simulink model "spc_nonlinear_observer_extended"  (R2022b)
settings: Solver=VariableStepAuto  StartTime=0.0  StopTime=30  RelTol=1e-3
undefined symbols (not defined in the file): A, B, C, D, g, Ki, Kp, L, l, M, m
settings Model: Creator=CANER  LastModifiedBy=CANER

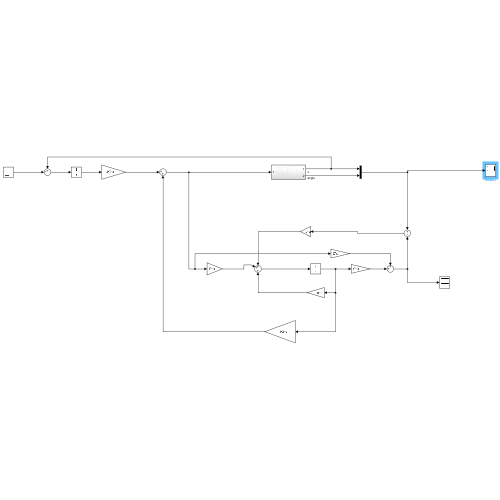
[thumbnail: Simulink's stored preview of the top-level diagram]
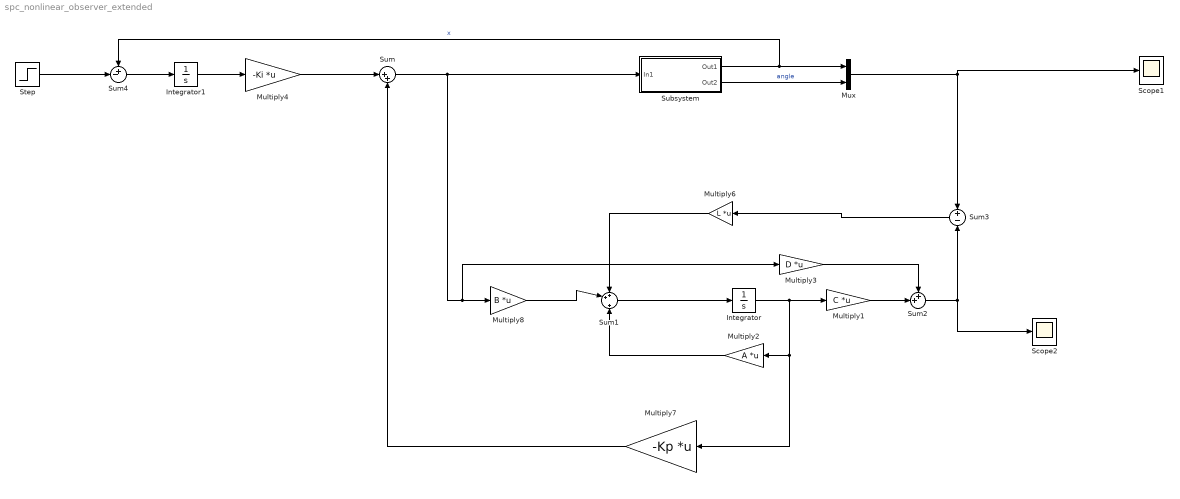
== system spc_nonlinear_observer_extended ==
  Integrator : Integrator
  Integrator1 : Integrator
  Multiply1 : Gain  Gain=C  Multiplication=Matrix(K*u)
  Multiply2 : Gain  Gain=A  Multiplication=Matrix(K*u)
  Multiply3 : Gain  Gain=D  Multiplication=Matrix(K*u)
  Multiply4 : Gain  Gain=-Ki  Multiplication=Matrix(K*u)
  Multiply6 : Gain  Gain=L  Multiplication=Matrix(K*u)
  Multiply7 : Gain  Gain=-Kp  Multiplication=Matrix(K*u)
  Multiply8 : Gain  Gain=B  Multiplication=Matrix(K*u)
  Mux : Mux  Inputs=2
  Scope1 : Scope
  Scope2 : Scope
  Step : Step  Time=0  SampleTime=0
  Subsystem : Subsystem
  Sum : Sum  Inputs=|++
  Sum1 : Sum  Inputs=++|+
  Sum2 : Sum  Inputs=++|
  Sum3 : Sum  Inputs=+|-
  Sum4 : Sum  Inputs=+-|
  wires:
  Multiply7/1 -> Sum/2
  Multiply6/1 -> Sum1/1
  Sum3/1 -> Multiply6/1
  Multiply8/1 -> Sum1/2
  Multiply2/1 -> Sum1/3
  Sum1/1 -> Integrator/1
  Integrator/1 -> Multiply7/1, Multiply2/1, Multiply1/1
  Sum2/1 -> Sum3/2, Scope2/1
  Sum/1 -> Subsystem/1(In1), Multiply3/1, Multiply8/1
  Subsystem/1(Out1) -> Sum4/1, Mux/1  "x"
  Multiply1/1 -> Sum2/2
  Multiply3/1 -> Sum2/1
  Mux/1 -> Sum3/1, Scope1/1
  Subsystem/2(Out2) -> Mux/2  "angle"
  Step/1 -> Sum4/2
  Multiply4/1 -> Sum/1
  Integrator1/1 -> Multiply4/1
  Sum4/1 -> Integrator1/1

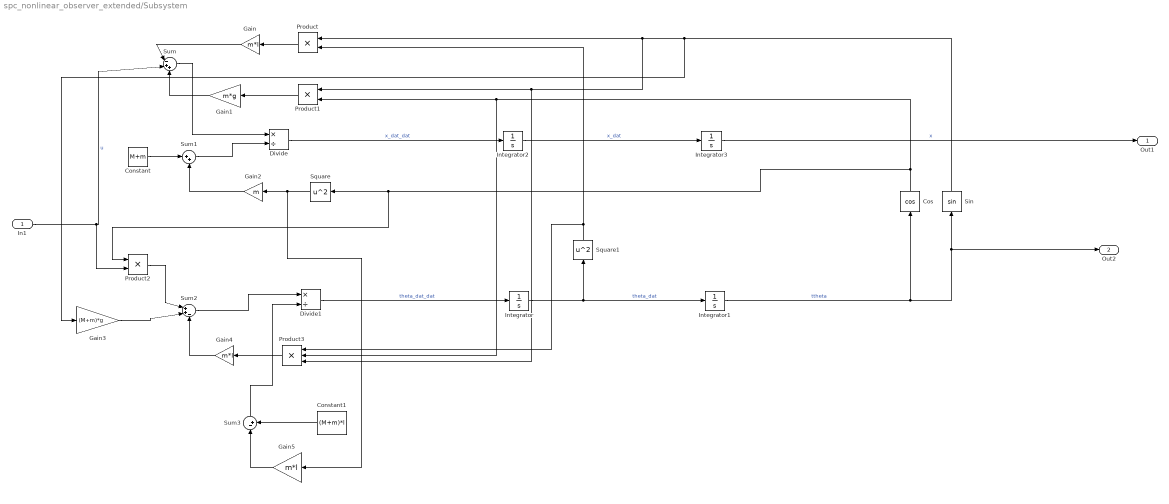
== system spc_nonlinear_observer_extended/Subsystem ==
  In1 : Inport
  Constant : Constant  Value=M+m
  Constant1 : Constant  Value=(M+m)*l
  Cos : Trigonometry  Operator=cos
  Divide : Product  Inputs=*/
  Divide1 : Product  Inputs=*/
  Gain : Gain  Gain=m*l
  Gain1 : Gain  Gain=m*g
  Gain2 : Gain  Gain=m
  Gain3 : Gain  Gain=(M+m)*g
  Gain4 : Gain  Gain=m*l
  Gain5 : Gain  Gain=m*l
  Integrator{,1..3} (4 alike) : Integrator
  Product : Product
  Product1 : Product
  Product2 : Product
  Product3 : Product  Inputs=3
  Sin : Trigonometry
  Square : Math  Operator=square
  Square1 : Math  Operator=square
  Sum : Sum  Inputs=|-++
  Sum1 : Sum  Inputs=|++
  Sum2 : Sum  Inputs=|++-
  Sum3 : Sum  Inputs=|-+
  Out1 : Outport
  Out2 : Outport  Port=2
  wires:
  Integrator/1 -> Integrator1/1, Square1/1  "theta_dat"
  Integrator2/1 -> Integrator3/1  "x_dat"
  Integrator3/1 -> Out1/1  "x"
  Divide/1 -> Integrator2/1  "x_dat_dat"
  Divide1/1 -> Integrator/1  "theta_dat_dat"
  Integrator1/1 -> Out2/1, Sin/1, Cos/1  "ttheta"
  In1/1 -> Product2/2, Sum/2  "u"
  Product/1 -> Gain/1
  Gain/1 -> Sum/1
  Gain1/1 -> Sum/3
  Cos/1 -> Product2/1, Square/1, Product3/2, Product1/2
  Product1/1 -> Gain1/1
  Sum/1 -> Divide/1
  Constant/1 -> Sum1/1
  Gain2/1 -> Sum1/2
  Square/1 -> Gain5/1, Gain2/1
  Sum1/1 -> Divide/2
  Product2/1 -> Sum2/1
  Sin/1 -> Gain3/1, Product3/3, Product1/1, Product/1
  Gain3/1 -> Sum2/2
  Gain4/1 -> Sum2/3
  Product3/1 -> Gain4/1
  Sum2/1 -> Divide1/1
  Constant1/1 -> Sum3/2
  Gain5/1 -> Sum3/1
  Sum3/1 -> Divide1/2
  Square1/1 -> Product3/1, Product/2
